simulink model "Nonlin_ve_Lin_Bir_Arada_Ters_Sarkac"  (R2022a)
settings: Solver=ode4  StartTime=0.0  StopTime=10.0  FixedStep=1/1000  RelTol=1e-3
InitFcn:
  | Sarkac_Parametrelerini_Yukle
values from neighbouring files (symbols this model uses):
  A = [0      1              0           0 ... (first row only)    [Sarkac_Parametrelerini_Yukle.m]
  b = 0.1    [Sarkac_Parametrelerini_Yukle.m]
  B = [     0 ... (first row only)    [Sarkac_Parametrelerini_Yukle.m]
  Baslangic_Degerleri = [0,0,pi,0]    [Sarkac_Parametrelerini_Yukle.m]
  Baslangic_Degerleri_Lin = [0,0,0,0]    [Sarkac_Parametrelerini_Yukle.m]
  C = [1 0 0 0 ... (first row only)    [Sarkac_Parametrelerini_Yukle.m]
  D = [0 ... (first row only)    [Sarkac_Parametrelerini_Yukle.m]
  g = 9.8    [Sarkac_Parametrelerini_Yukle.m]
  I = 0.006    [Sarkac_Parametrelerini_Yukle.m]
  l = 0.3    [Sarkac_Parametrelerini_Yukle.m]
  M = 0.5    [Sarkac_Parametrelerini_Yukle.m]
  m = 0.2    [Sarkac_Parametrelerini_Yukle.m]
undefined symbols (not defined in the file or in its folder): sigbuilder_block
libraries: vrlib x2
settings Model: Creator=Fatabi  LastModifiedBy=Fatabi
settings SolverCC: AlgebraicLoopSolver=TrustRegion
settings DebuggingCC: UnconnectedInputMsg=warning  UnconnectedOutputMsg=warning  UnconnectedLineMsg=warning  SFMachineParentedDataDiag=warning

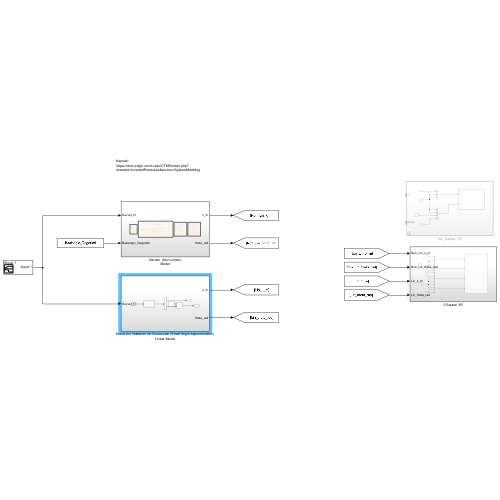
[thumbnail: Simulink's stored preview of the top-level diagram]
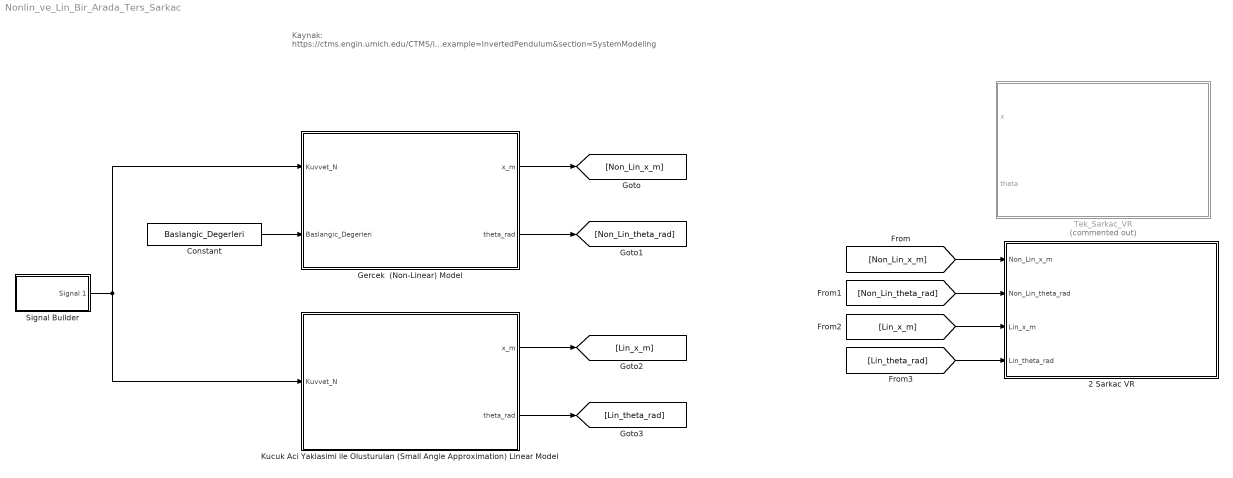
== system Nonlin_ve_Lin_Bir_Arada_Ters_Sarkac ==
  note: Kaynak:
      | https://ctms.engin.umich.edu/CTMS/index.php?example=InvertedPendulum&section=SystemModeling
  2 Sarkac VR : Subsystem
  Constant : Constant  Value=Baslangic_Degerleri
  Gercek  (Non-Linear) Model : Subsystem
  Kucuk Aci Yaklasimi ile Olusturulan (Small Angle Approximation) Linear Model : Subsystem
  Signal Builder : Subsystem  Tag=STV Subsys  LoadFcn=sigbuilder_block('load');  StartFcn=sigbuilder_block('start');  StopFcn=sigbuilder_block('stop');  ClipboardFcn=sigbuilder_block('clipboard');  mask(Sigbuilder block){tuvar=[0:10]}
      mask help: Simulink:masks:SigbuilderBlock_MD
      mask init:
      | if ~strcmp(get_param(bdroot(gcbh),'SimulationStatus'),'stopped') tuvar = sigbuilder_block('maskInit'); end
      settings: CopyFcn=sigbuilder_block('copy');  DeleteFcn=sigbuilder_block('delete');  ModelCloseFcn=sigbuilder_block('modelClose');  PreSaveFcn=sigbuilder_block('preSave');  PauseFcn=sigbuilder_block('pause');  ContinueFcn=sigbuilder_block('continue');  NameChangeFcn=sigbuilder_block('namechange');  OpenFcn=sigbuilder_block('open',[338.25 225.75 550.5 399.75 ]);  CloseFcn=sigbuilder_block('close');
      mask Display: plot(0, 0, 100, 100,[2, 2, 32, 32, 2], [68, 8, 8, 68, 68],[32, 2], [38, 38], [32, 19, 2],[53, 60, 44], [32, 17, 17, 2],[16, 16, 31, 31]);txt = getActiveGroup(gcbh);text(2, 100, txt,'verticalAlignment', 'top');
  "Tek_Sarkac_VR " : Subsystem  Commented=on
  wires:
  Signal Builder/1(Signal 1) -> Kucuk Aci Yaklasimi ile Olusturulan (Small Angle Approximation) Linear Model/1(Kuvvet_N), Gercek  (Non-Linear) Model/1(Kuvvet_N)
  Constant/1 -> Gercek  (Non-Linear) Model/2(Baslangic_Degerleri)
  Gercek  (Non-Linear) Model/1(x_m) -> [Non_Lin_x_m]
  Gercek  (Non-Linear) Model/2(theta_rad) -> [Non_Lin_theta_rad]
  Kucuk Aci Yaklasimi ile Olusturulan (Small Angle Approximation) Linear Model/1(x_m) -> [Lin_x_m]
  Kucuk Aci Yaklasimi ile Olusturulan (Small Angle Approximation) Linear Model/2(theta_rad) -> [Lin_theta_rad]
  [Non_Lin_x_m] -> 2 Sarkac VR/1(Non_Lin_x_m)
  [Non_Lin_theta_rad] -> 2 Sarkac VR/2("Non_Lin_theta_rad ")
  [Lin_x_m] -> 2 Sarkac VR/3(Lin_x_m)
  [Lin_theta_rad] -> 2 Sarkac VR/4(Lin_theta_rad)

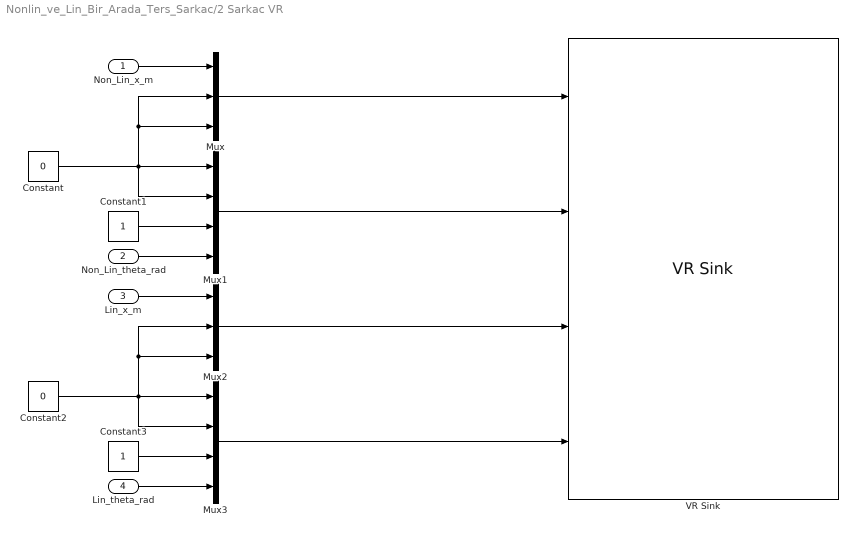
== system Nonlin_ve_Lin_Bir_Arada_Ters_Sarkac/2 Sarkac VR ==
  Non_Lin_x_m : Inport
  "Non_Lin_theta_rad " : Inport  Port=2
  Lin_x_m : Inport  Port=3
  Lin_theta_rad : Inport  Port=4
  Constant : Constant  Value=0
  Constant1 : Constant
  Constant2 : Constant  Value=0
  Constant3 : Constant
  Mux : Mux  Inputs=3
  Mux1 : Mux
  Mux2 : Mux  Inputs=3
  Mux3 : Mux
  VR Sink : vrlib/VR Sink  InstantiateOnLoad=on  SampleTime=0.02  ViewEnable=on  RemoteChange=off  RemoteView=off  FieldsWritten=Non_Lin_Araba.translation.3.1.1.double#Sarkac_Mentesesi.rotation.4.1.1.double#Lin_Araba.translation.3.1.1.double#Sarkac_Mentesesi_Lin.rotation.4.1.1.double  WorldFileName=NonLin_ve_Lin.wrl  AutoView=off  VideoDimensions=[]  AllowVariableSize=off  FigureProperties="{'Position', 'Name', 'Viewpoint', 'CameraBound', 'CameraDirection', 'CameraPosition', 'CameraUpVector', 'ZoomFactor', 'Antialiasing', 'Headlight', 'Lighting', 'NavPanel', 'Sound', 'StatusBar', 'Stereo3D', 'Stereo3DCameraOffset', 'Stereo3DHIT', 'ToolBar', 'Textures', 'Transparency', 'Triad', 'Wireframe', 'NavZones', 'NavMode', 'NavSpeed', 'CaptureFileFormat', 'CaptureFileName', 'Record2DCompressMethod', 'Record2DCompressQuality', 'Record2D', 'Record2DFileName', 'Record2DFPS'; [6.4000000000000000e+01   7.6000000000000000e+01   1.8570000000000000e+03   9.5300000000000000e+02], '', '_untitled_1', 'on', [0.0000000000000000e+00   0.0000000000000000e+00  -1.0000000000000000e+00], [0.0000000000000000e+00   0.0000000000000000e+00   0.0000000000000000e+00], [0.0000000000000000e+00   1.0000000000000000e+00   0.0000000000000000e+00], [1.0000000000000000e+00], 'on', 'on', 'on', 'halfbar', 'on', 'on', 'off', [1.0000000149011612e-01], [0.0000000000000000e+00], 'on', 'on', 'on', 'topleft', 'off', 'off', 'fly', 'normal', 'tif', '%f_anim_%n.tif', 'auto', [7.5000000000000000e+01], 'off', '%f_anim_%n.avi', 'auto'}"
  wires:
  Constant1/1 -> Mux1/3
  "Non_Lin_theta_rad "/1 -> Mux1/4
  Constant/1 -> Mux1/2, Mux/2, Mux/3, Mux1/1
  Non_Lin_x_m/1 -> Mux/1
  Mux/1 -> VR Sink/1
  Mux1/1 -> VR Sink/2
  Mux3/1 -> VR Sink/4
  Mux2/1 -> VR Sink/3
  Lin_x_m/1 -> Mux2/1
  Constant2/1 -> Mux3/1, Mux2/3, Mux2/2, Mux3/2
  Lin_theta_rad/1 -> Mux3/4
  Constant3/1 -> Mux3/3

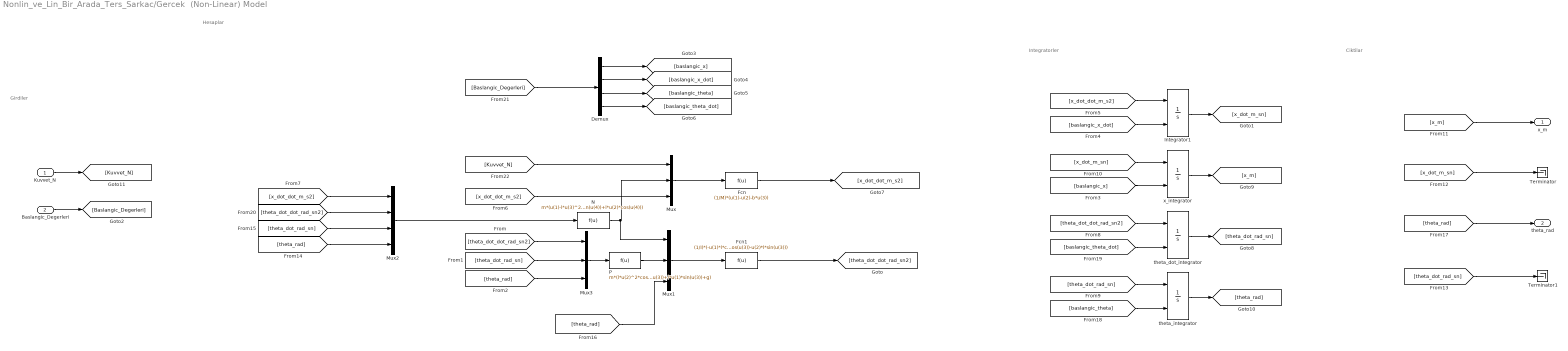
== system Nonlin_ve_Lin_Bir_Arada_Ters_Sarkac/Gercek  (Non-Linear) Model ==
  note: Integratorler
  note: Girdiler
  note: Ciktilar
  note: Hesaplar
  Kuvvet_N : Inport
  Baslangic_Degerleri : Inport  Port=2
  Demux : Demux
  Fcn : Fcn  Expr=(1/M)*(u(1)-u(2)-b*u(3))
  Fcn1 : Fcn  Expr=(1/I)*(-u(1)*l*cos(u(3))-u(2)*l*sin(u(3)))
  Integrator1 : Integrator  InitialConditionSource=external  ContinuousStateAttributes='x_dot_m_sn'
  Mux : Mux  Inputs=3
  Mux1 : Mux  Inputs=3
  Mux2 : Mux
  Mux3 : Mux  Inputs=3
  N : Fcn  Expr=m*(u(1)-l*u(3)^2*sin(u(4))+l*u(2)*cos(u(4)))
  P : Fcn  Expr=m*(l*u(2)^2*cos(u(3))+l*u(1)*sin(u(3))+g)
  Terminator : Terminator
  Terminator1 : Terminator
  theta_dot_integrator : Integrator  InitialConditionSource=external  ContinuousStateAttributes='theta_dot_rad_sn'
  theta_integrator : Integrator  InitialConditionSource=external  InitialCondition=pi-0.1  ContinuousStateAttributes='theta_rad'
  x_integrator : Integrator  InitialConditionSource=external  ContinuousStateAttributes='x_m'
  x_m : Outport
  theta_rad : Outport  Port=2
  wires:
  [x_dot_dot_m_s2] -> Mux/3
  Fcn/1 -> [x_dot_dot_m_s2]
  [Kuvvet_N] -> Mux/1
  N/1 -> Mux1/1, Mux/2
  Mux/1 -> Fcn/1
  Fcn1/1 -> [theta_dot_dot_rad_sn2]
  Mux1/1 -> Fcn1/1
  P/1 -> Mux1/2
  Mux2/1 -> N/1
  [theta_dot_dot_rad_sn2] -> Mux3/1
  [theta_dot_rad_sn] -> Mux3/2
  [theta_rad] -> Mux3/3
  Mux3/1 -> P/1
  [Baslangic_Degerleri] -> Demux/1
  Demux/1 -> [baslangic_x]
  Demux/2 -> [baslangic_x_dot]
  Demux/3 -> [baslangic_theta]
  Demux/4 -> [baslangic_theta_dot]
  [baslangic_x] -> x_integrator/2
  x_integrator/1 -> [x_m]
  [baslangic_x_dot] -> Integrator1/2
  [x_dot_dot_m_s2] -> Integrator1/1
  Integrator1/1 -> [x_dot_m_sn]
  [x_dot_dot_m_s2] -> Mux2/1
  [theta_dot_dot_rad_sn2] -> theta_dot_integrator/1
  theta_dot_integrator/1 -> [theta_dot_rad_sn]
  [x_dot_m_sn] -> x_integrator/1
  [x_m] -> x_m/1
  [x_dot_m_sn] -> Terminator/1
  [theta_dot_rad_sn] -> theta_integrator/1
  theta_integrator/1 -> [theta_rad]
  [theta_rad] -> Mux2/4
  [theta_dot_rad_sn] -> Mux2/3
  [theta_rad] -> Mux1/3
  [theta_rad] -> theta_rad/1
  [baslangic_theta] -> theta_integrator/2
  [baslangic_theta_dot] -> theta_dot_integrator/2
  [theta_dot_dot_rad_sn2] -> Mux2/2
  Baslangic_Degerleri/1 -> [Baslangic_Degerleri]
  Kuvvet_N/1 -> [Kuvvet_N]
  [theta_dot_rad_sn] -> Terminator1/1

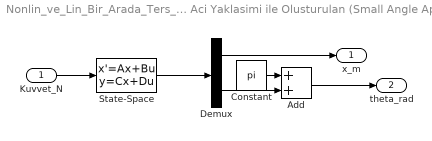
== system Nonlin_ve_Lin_Bir_Arada_Ters_Sarkac/Kucuk Aci Yaklasimi ile Olusturulan (Small Angle Approximation) Linear Model ==
  Kuvvet_N : Inport
  Add : Sum
  Constant : Constant  Value=pi
  Demux : Demux  Outputs=2
  State-Space : StateSpace  A=A  B=B  C=C  D=D  InitialCondition=Baslangic_Degerleri_Lin
  x_m : Outport
  theta_rad : Outport  Port=2
  wires:
  State-Space/1 -> Demux/1
  Demux/1 -> x_m/1
  Demux/2 -> Add/2
  Kuvvet_N/1 -> State-Space/1
  Add/1 -> theta_rad/1
  Constant/1 -> Add/1

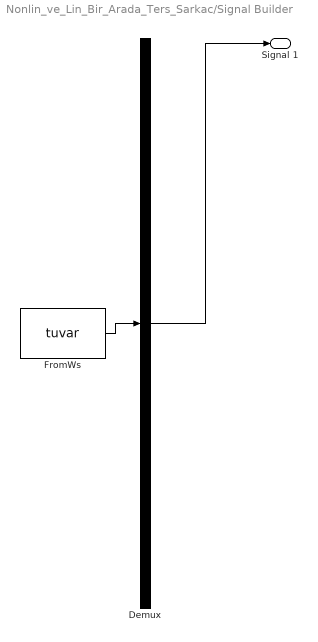
== system Nonlin_ve_Lin_Bir_Arada_Ters_Sarkac/Signal Builder ==
  Demux : Demux  Tag=STV Demux  Outputs=1
      settings: DisplayOption=none
  FromWs : FromWorkspace  Tag=STV FromWs  VariableName=tuvar
      SigBuilderData=|
      | common.afterFinalStr = 'Extrapolate'
      | common.sampleTime = 0
      | dataSet.timeRange = [0 10]
      | dataSet.name = 'Group 1'
      | sbobj.Groups.Name = 'Group 1'
      | sbobj.Groups.Signals.Name = 'Signal 1'
      | sbobj.Groups.Signals.XData = [0 1 1 1.5 1.5 10]
      | sbobj.Groups.Signals.YData = [0 0 1 1 0 0]
  Signal 1 : Outport  Tag=STV Outport
  wires:
  Demux/1 -> Signal 1/1
  FromWs/1 -> Demux/1

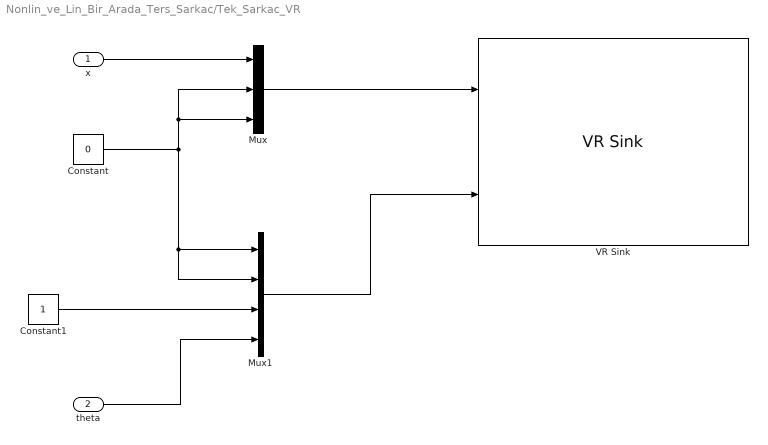
== system Nonlin_ve_Lin_Bir_Arada_Ters_Sarkac/Tek_Sarkac_VR  ==
  x : Inport
  "theta " : Inport  Port=2
  Constant : Constant  Value=0
  Constant1 : Constant
  Mux : Mux  Inputs=3
  Mux1 : Mux
  VR Sink : vrlib/VR Sink  InstantiateOnLoad=on  SampleTime=0.02  ViewEnable=on  RemoteChange=off  RemoteView=off  FieldsWritten=Kutu.translation.3.1.1.double#Mentese1.rotation.4.1.1.double  WorldFileName=sarkac.wrl  AutoView=off  VideoDimensions=[]  AllowVariableSize=off
  wires:
  x/1 -> Mux/1
  Constant/1 -> Mux/3, Mux/2, Mux1/2, Mux1/1
  "theta "/1 -> Mux1/4
  Constant1/1 -> Mux1/3
  Mux/1 -> VR Sink/1
  Mux1/1 -> VR Sink/2
